simulink model "Colin_C_1_2020b"  (Simulink 10.3)
settings: Solver=ode45  StartTime=0.0  StopTime=5  RelTol=1e-3  AbsTol=1e-4
undefined symbols (not defined in the file or in its folder): C3, pendubot_eqt, Ts
libraries: simulink x4, SignalEditorBlockLib x1
Description:
  | Non-linear mathematical model of pendubot electro-mechanical system (underactuated pendulum system).
settings Model: Creator=Hynek Prochazka  LastModifiedBy=Colin  ExtModeTrigMode=oneshot  ExtModeArmWhenConnect=off
settings SolverCC: AutoScaleAbsTol=off
settings DataIOCC: SaveOutput=off
settings OptimizationCC: BlockReduction=off  BooleanDataType=off
settings DebuggingCC: SaveWithParameterizedLinksMsg=none  SignalResolutionControl=TryResolveAllWithWarning  MultiTaskDSMMsg=warning  MultiTaskCondExecSysMsg=none
settings HardwareCC: TargetUnknown=on
settings RTWCC: TemplateMakefile=grt_unix.tmf
settings ConfigComp: CovSFcnEnable=off

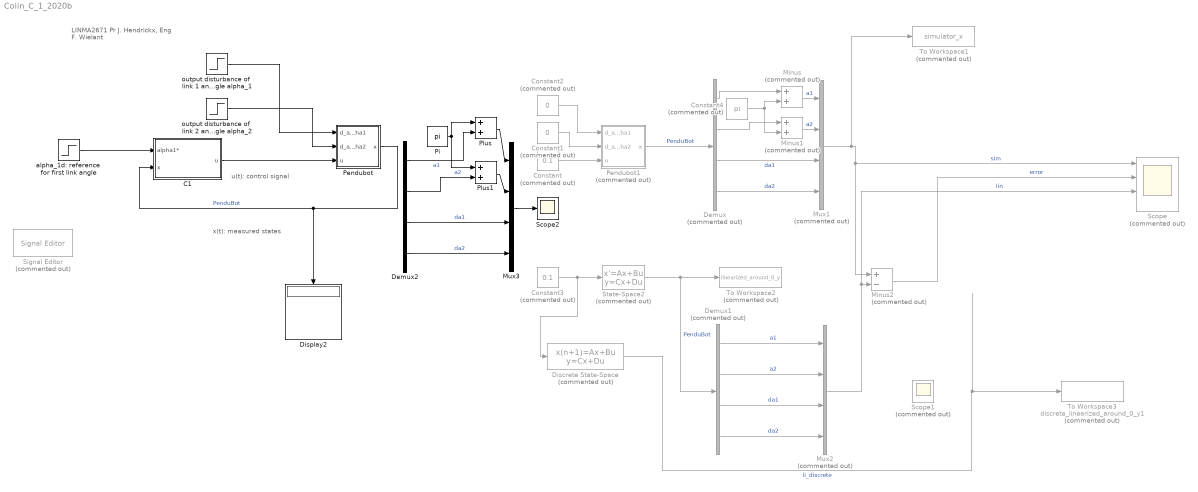
== system Colin_C_1_2020b ==
  note: u(t):
      | control signal
  note: x(t): measured states
  note: LINMA2671
      | Pr J. Hendrickx, Eng F. Wielant
  C1 : Subsystem
  Constant : Constant  Commented=on  Value=0.1
  Constant1 : Constant  Commented=on  Value=0
  Constant2 : Constant  Commented=on  Value=0
  Constant3 : Constant  Commented=on  Value=0.1
  Constant4 : Constant  Commented=on  Value=pi
  Demux : Demux  Commented=on
      settings: DisplayOption=none
  Demux1 : Demux  Commented=on
      settings: DisplayOption=none
  Demux2 : Demux
      settings: DisplayOption=none
  Discrete State-Space : DiscreteStateSpace  Commented=on  A=[0.9993,0.0004,0.004,0;0.0014,0.9987,0,0.004;-0.3693,0.2122,0.9993,0.0004;0.7023,-0.6366,0.0014,0.9987]  B=[0.0004;-0.0007;0.1859;-0.3535]  C=eye(4)  D=[0;0;0;0]  SampleTime=Ts
  Display2 : Display
  Minus : Sum  Commented=on
  Minus1 : Sum  Commented=on
  Minus2 : Sum  Commented=on  Inputs=+-
  Mux1 : Mux  Commented=on
  Mux2 : Mux  Commented=on
  Mux3 : Mux
  Pendubot : Subsystem  mask(Pendubot){x10=0, x20=0, x30=0, x40=0, Ts=Ts}
      mask prompts: x10 "Initial angle of link 1:"; x20 "Initial angular speed for link 1 :"; x30 "Initial angle of link 2 :"; x40 "Initial angular speed for link 2 :"; Ts "Sampling time [s] :"
      mask help: Initial conditions (initial state)
      mask Display:
      | plot(0.1*[1 9],0.1*[1 1])
      | plot(0.1*[1.5 1.5 8.5 8.5],0.1*[1 4 4 1])
      | plot(0.1*[5.2 8.2],0.1*[1 5])
      | plot(0.1*[4.8 7.8],0.1*[1 5])
      | plot(0.1*[7.8 5.8],0.1*[5 9.5])
      | plot(0.1*[8.2 6.2],0.1*[5 9.5])
  Pendubot1 : Subsystem  Commented=on  mask(Pendubot){x10=4*pi/5, x20=0, x30=pi, x40=0, Ts=Ts}
      mask prompts: x10 "Initial angle of link 1:"; x20 "Initial angular speed for link 1 :"; x30 "Initial angle of link 2 :"; x40 "Initial angular speed for link 2 :"; Ts "Sampling time [s] :"
      mask help: Initial conditions (initial state)
      mask Display:
      | plot(0.1*[1 9],0.1*[1 1])
      | plot(0.1*[1.5 1.5 8.5 8.5],0.1*[1 4 4 1])
      | plot(0.1*[5.2 8.2],0.1*[1 5])
      | plot(0.1*[4.8 7.8],0.1*[1 5])
      | plot(0.1*[7.8 5.8],0.1*[5 9.5])
      | plot(0.1*[8.2 6.2],0.1*[5 9.5])
  Pi : Constant  Value=pi  OutDataTypeStr=Inherit: Inherit via back propagation
  Plus : Sum
  Plus1 : Sum
  Scope : Scope  Commented=on  NumInputPorts=4
  Scope1 : Scope  Commented=on
  Scope2 : Scope
  Signal Editor : SignalEditorBlockLib/Signal Editor  Commented=on  FileName=untitled.mat  ActiveScenario=Scenario  ActiveSignal=Signal 1  IsBus=off  OutputBusObjectStr=Bus: BusObject  SampleTime=0  Interpolate=off  ZeroCross=off  OutputAfterFinalValue=Setting to zero  Unit=inherit  PreserveSignalName=on
  State-Space2 : StateSpace  Commented=on  A=[0,0,1,0;0,0,0,1;57.9843,-34.6580,0,0;-87.489,105.4244,0,0]  B=[0;0;40.9835;-70.8893]  C=eye(4)  D=[0;0;0;0]  InitialCondition=[0;0;0;0]
  To Workspace1 : ToWorkspace  Commented=on  VariableName=simulator_x  SaveFormat=Timeseries  SampleTime=Ts
  To Workspace2 : ToWorkspace  Commented=on  VariableName=linearized_around_0_y  SaveFormat=Timeseries  SampleTime=Ts
  To Workspace3 : ToWorkspace  Commented=on  VariableName=discrete_linearized_around_0_y1  SaveFormat=Timeseries  SampleTime=Ts
  "alpha_1d: reference  for first link angle " : Step  Time=2  After=4*pi/5  SampleTime=Ts
  output disturbance of  link 1 angle alpha_1 : Step  Time=5  After=0  SampleTime=Ts
  output disturbance of  link 2 angle alpha_2 : Step  Time=2  After=0  SampleTime=Ts
  wires:
  Pendubot/1(x) -> Display2/1, C1/2(x)  "PenduBot"
  C1/1(u) -> Pendubot/3(u)
  Constant/1 -> Pendubot1/3(u)
  Constant2/1 -> Pendubot1/1(d_alpha1)
  Constant1/1 -> Pendubot1/2(d_alpha2)
  Pendubot1/1(x) -> Demux/1  "PenduBot"
  Constant3/1 -> State-Space2/1, Discrete State-Space/1
  Minus/1 -> Mux1/1  "a1"
  Demux/1 -> Minus/1
  Constant4/1 -> Minus1/2, Minus/2
  Minus1/1 -> Mux1/2  "a2"
  Demux/2 -> Minus1/1
  Demux/3 -> Mux1/3  "da1"
  Demux/4 -> Mux1/4  "da2"
  Mux1/1 -> To Workspace1/1, Minus2/1, Scope/1  "sim"
  Demux1/2 -> Mux2/2  "a2"
  Demux1/1 -> Mux2/1  "a1"
  State-Space2/1 -> Demux1/1, To Workspace2/1  "PenduBot"
  Demux1/4 -> Mux2/4  "da2"
  Mux2/1 -> Minus2/2, Scope/3  "lin"
  Demux1/3 -> Mux2/3  "da1"
  Minus2/1 -> Scope/2  "error"
  Discrete State-Space/1 -> To Workspace3/1  "li_discrete"
  output disturbance of  link 1 angle alpha_1/1 -> Pendubot/1(d_alpha1)
  output disturbance of  link 2 angle alpha_2/1 -> Pendubot/2(d_alpha2)
  "alpha_1d: reference  for first link angle "/1 -> C1/1(alpha1*)
  Demux2/3 -> Mux3/3  "da1"
  Demux2/2 -> Plus1/2  "a2"
  Demux2/4 -> Mux3/4  "da2"
  Demux2/1 -> Plus/2  "a1"
  Mux3/1 -> Scope2/1
  Plus/1 -> Mux3/1
  Pi/1 -> Plus1/1, Plus/1
  Plus1/1 -> Mux3/2

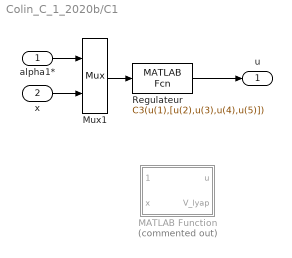
== system Colin_C_1_2020b/C1 ==
  alpha1* : Inport
  x : Inport  Port=2
  MATLAB Function : MATLAB Function  Commented=on  TreatAsAtomicUnit=on
  Mux1 : Mux  Inputs=2
  Regulateur : MATLABFcn  MATLABFcn=C3(u(1),[u(2),u(3),u(4),u(5)])
  u : Outport
  wires:
  Mux1/1 -> Regulateur/1
  alpha1*/1 -> Mux1/1
  x/1 -> Mux1/2
  Regulateur/1 -> u/1

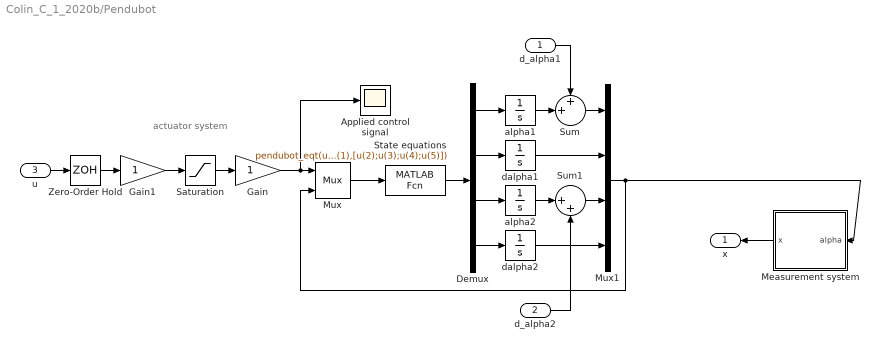
== system Colin_C_1_2020b/Pendubot ==
  note: actuator system
  d_alpha1 : Inport
  d_alpha2 : Inport  Port=2
  u : Inport  Port=3
  Applied control signal : Scope
  Demux : Demux
      settings: DisplayOption=none
  Gain : Gain  SaturateOnIntegerOverflow=on  OutDataTypeStr=Inherit: Same as input  ParamDataTypeStr=Inherit: Same as input
  Gain1 : Gain  SaturateOnIntegerOverflow=on  OutDataTypeStr=Inherit: Same as input  ParamDataTypeStr=Inherit: Same as input
  Measurement system : Subsystem
  Mux : Mux  Inputs=2
  Mux1 : Mux
  Saturation : Saturate  UpperLimit=10  LowerLimit=-10
  State equations : MATLABFcn  MATLABFcn=pendubot_eqt(u(1),[u(2);u(3);u(4);u(5)])  OutputDimensions=4
  Sum : Sum  Inputs=++|  InputSameDT=on  SaturateOnIntegerOverflow=on  OutDataTypeStr=Inherit: Same as first input
  Sum1 : Sum  Inputs=|++  InputSameDT=on  SaturateOnIntegerOverflow=on  OutDataTypeStr=Inherit: Same as first input
  Zero-Order Hold : ZeroOrderHold  SampleTime=Ts
  alpha1 : Integrator  InitialCondition=x10
  alpha2 : Integrator  InitialCondition=x30
  dalpha1 : Integrator  InitialCondition=x20
  dalpha2 : Integrator  InitialCondition=x40
  x : Outport
  wires:
  u/1 -> Zero-Order Hold/1
  State equations/1 -> Demux/1
  Mux/1 -> State equations/1
  Saturation/1 -> Gain/1
  Zero-Order Hold/1 -> Gain1/1
  Gain1/1 -> Saturation/1
  Gain/1 -> Mux/1, Applied control signal/1
  Mux1/1 -> Mux/2, Measurement system/1(alpha)
  dalpha2/1 -> Mux1/4
  Demux/1 -> alpha1/1
  Demux/2 -> dalpha1/1
  Demux/3 -> alpha2/1
  Demux/4 -> dalpha2/1
  Sum/1 -> Mux1/1
  Sum1/1 -> Mux1/3
  dalpha1/1 -> Mux1/2
  alpha1/1 -> Sum/2
  d_alpha1/1 -> Sum/1
  alpha2/1 -> Sum1/1
  d_alpha2/1 -> Sum1/2
  Measurement system/1(x) -> x/1

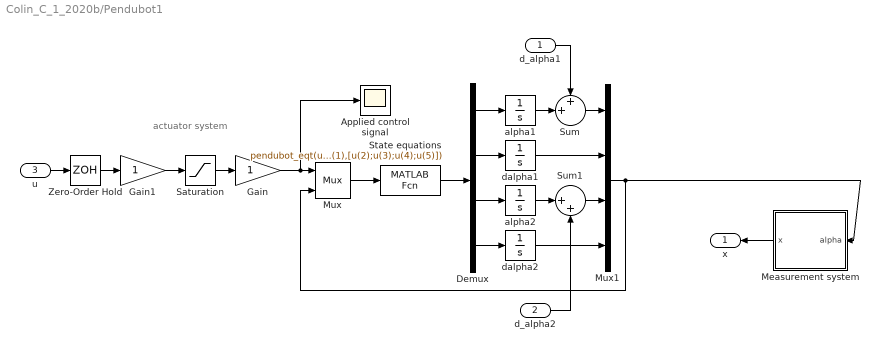
== system Colin_C_1_2020b/Pendubot1 ==
  note: actuator system
  d_alpha1 : Inport
  d_alpha2 : Inport  Port=2
  u : Inport  Port=3
  Applied control signal : Scope
  Demux : Demux
      settings: DisplayOption=none
  Gain : Gain  SaturateOnIntegerOverflow=on  OutDataTypeStr=Inherit: Same as input  ParamDataTypeStr=Inherit: Same as input
  Gain1 : Gain  SaturateOnIntegerOverflow=on  OutDataTypeStr=Inherit: Same as input  ParamDataTypeStr=Inherit: Same as input
  Measurement system : Subsystem
  Mux : Mux  Inputs=2
  Mux1 : Mux
  Saturation : Saturate  UpperLimit=10  LowerLimit=-10
  State equations : MATLABFcn  MATLABFcn=pendubot_eqt(u(1),[u(2);u(3);u(4);u(5)])  OutputDimensions=4
  Sum : Sum  Inputs=++|  InputSameDT=on  SaturateOnIntegerOverflow=on  OutDataTypeStr=Inherit: Same as first input
  Sum1 : Sum  Inputs=|++  InputSameDT=on  SaturateOnIntegerOverflow=on  OutDataTypeStr=Inherit: Same as first input
  Zero-Order Hold : ZeroOrderHold  SampleTime=Ts
  alpha1 : Integrator  InitialCondition=x10
  alpha2 : Integrator  InitialCondition=x30
  dalpha1 : Integrator  InitialCondition=x20
  dalpha2 : Integrator  InitialCondition=x40
  x : Outport
  wires:
  u/1 -> Zero-Order Hold/1
  State equations/1 -> Demux/1
  Mux/1 -> State equations/1
  Saturation/1 -> Gain/1
  Zero-Order Hold/1 -> Gain1/1
  Gain1/1 -> Saturation/1
  Gain/1 -> Mux/1, Applied control signal/1
  Mux1/1 -> Mux/2, Measurement system/1(alpha)
  dalpha2/1 -> Mux1/4
  Demux/1 -> alpha1/1
  Demux/2 -> dalpha1/1
  Demux/3 -> alpha2/1
  Demux/4 -> dalpha2/1
  Sum/1 -> Mux1/1
  Sum1/1 -> Mux1/3
  dalpha1/1 -> Mux1/2
  alpha1/1 -> Sum/2
  d_alpha1/1 -> Sum/1
  alpha2/1 -> Sum1/1
  d_alpha2/1 -> Sum1/2
  Measurement system/1(x) -> x/1

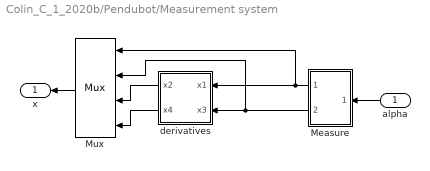
== system Colin_C_1_2020b/Pendubot/Measurement system ==
  alpha : Inport
  Measure : Subsystem
  Mux : Mux
  derivatives : Subsystem
  x : Outport
  wires:
  derivatives/2(x4) -> Mux/4
  Mux/1 -> x/1
  Measure/1(xm(1)) -> derivatives/1(x1), Mux/1
  alpha/1 -> Measure/1(alpha)
  Measure/2(xm(1)1) -> derivatives/2(x3), Mux/2
  derivatives/1(x2) -> Mux/3

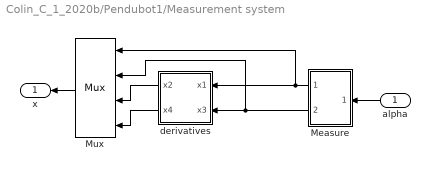
== system Colin_C_1_2020b/Pendubot1/Measurement system ==
  alpha : Inport
  Measure : Subsystem
  Mux : Mux
  derivatives : Subsystem
  x : Outport
  wires:
  derivatives/2(x4) -> Mux/4
  Mux/1 -> x/1
  Measure/1(xm(1)) -> derivatives/1(x1), Mux/1
  alpha/1 -> Measure/1(alpha)
  Measure/2(xm(1)1) -> derivatives/2(x3), Mux/2
  derivatives/1(x2) -> Mux/3

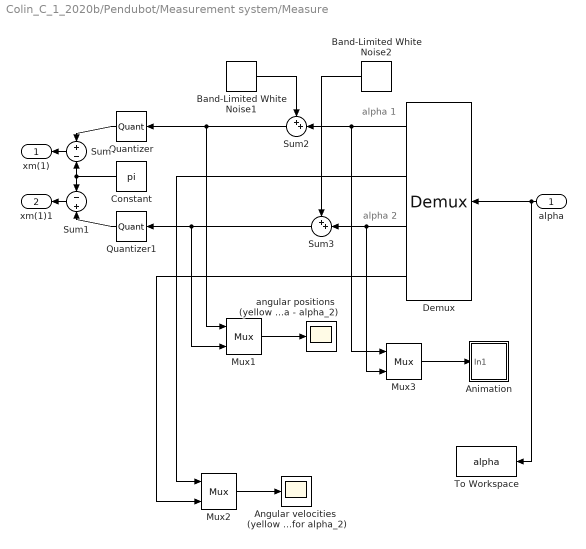
== system Colin_C_1_2020b/Pendubot/Measurement system/Measure ==
  note: alpha 1
  note: alpha 2
  alpha : Inport
  "Angular velocities  (yellow - for alpha_1,  magenta - for alpha_2) " : Scope
  Animation : Subsystem  mask(Animation Block){ts=10*0.003}
      mask prompts: ts "Sample time:"
      mask Display: plot([.1,.9],[.9,.9],[.5,.2],[.9,.25],[.475,.475,.525,.525,.475],[.875,.925,.925,.875,.875])
  Band-Limited White Noise1 : simulink/Sources/Band-Limited White Noise  Cov=[1e-8]  Ts=Ts  seed=[23341]
  Band-Limited White Noise2 : simulink/Sources/Band-Limited White Noise  Cov=[1e-7]  Ts=Ts  seed=[32214]
  Constant : Constant  Value=pi
  Demux : Demux
      settings: DisplayOption=none
  Mux1 : Mux  Inputs=2
  Mux2 : Mux  Inputs=2
  Mux3 : Mux  Inputs=2
  Quantizer : Quantizer  QuantizationInterval=2*pi/5000
  Quantizer1 : Quantizer  QuantizationInterval=2*pi/5000
  Sum : Sum  Inputs=+-  InputSameDT=on  SaturateOnIntegerOverflow=on  OutDataTypeStr=Inherit: Same as first input
  Sum1 : Sum  Inputs=-+  InputSameDT=on  SaturateOnIntegerOverflow=on  OutDataTypeStr=Inherit: Same as first input
  Sum2 : Sum  Inputs=++|  InputSameDT=on  SaturateOnIntegerOverflow=on  OutDataTypeStr=Inherit: Same as first input
  Sum3 : Sum  Inputs=++|  InputSameDT=on  SaturateOnIntegerOverflow=on  OutDataTypeStr=Inherit: Same as first input
  To Workspace : ToWorkspace  VariableName=alpha  SampleTime=Ts
  "angular positions  (yellow - alpha_1,  magenta - alpha_2)" : Scope
  xm(1) : Outport  Tag=alpha1
  xm(1)1 : Outport  Port=2
  wires:
  alpha/1 -> To Workspace/1, Demux/1
  Demux/2 -> Mux2/1
  Demux/4 -> Mux2/2
  Mux2/1 -> "Angular velocities  (yellow - for alpha_1,  magenta - for alpha_2) "/1
  Sum/1 -> xm(1)/1
  Quantizer/1 -> Sum/1
  Sum1/1 -> xm(1)1/1
  Quantizer1/1 -> Sum1/2
  Constant/1 -> Sum/2, Sum1/1
  Band-Limited White Noise1/1 -> Sum2/1
  Band-Limited White Noise2/1 -> Sum3/1
  Sum2/1 -> Quantizer/1, Mux1/1
  Sum3/1 -> Quantizer1/1, Mux1/2
  Mux1/1 -> "angular positions  (yellow - alpha_1,  magenta - alpha_2)"/1
  Demux/1 -> Sum2/2, Mux3/1
  Demux/3 -> Sum3/2, Mux3/2
  Mux3/1 -> Animation/1(In1)

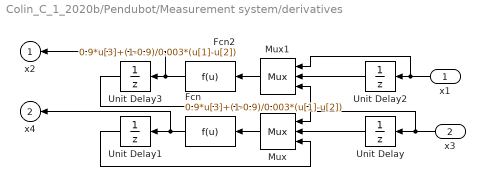
== system Colin_C_1_2020b/Pendubot/Measurement system/derivatives ==
  x1 : Inport
  x3 : Inport  Port=2
  Fcn : Fcn  Expr=0.9*u[3]+(1-0.9)/0.003*(u[1]-u[2])
  Fcn2 : Fcn  Expr=0.9*u[3]+(1-0.9)/0.003*(u[1]-u[2])
  Mux : Mux  Inputs=3
  Mux1 : Mux  Inputs=3
  Unit Delay{,1..3} (4 alike) : UnitDelay  SampleTime=Ts  HasFrameUpgradeWarning=on
  x2 : Outport
  x4 : Outport  Port=2
  wires:
  Unit Delay/1 -> Mux/2
  Mux/1 -> Fcn/1
  Unit Delay1/1 -> Mux/3
  Fcn/1 -> Unit Delay1/1, x4/1
  x3/1 -> Unit Delay/1, Mux/1
  Unit Delay2/1 -> Mux1/2
  Mux1/1 -> Fcn2/1
  Unit Delay3/1 -> Mux1/3
  x1/1 -> Unit Delay2/1, Mux1/1
  Fcn2/1 -> Unit Delay3/1, x2/1

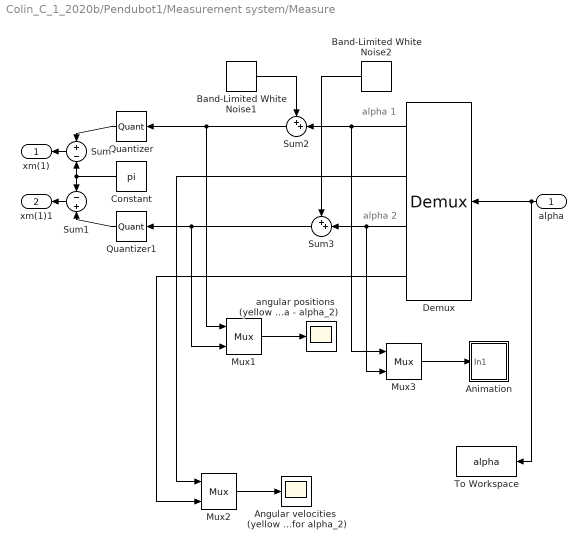
== system Colin_C_1_2020b/Pendubot1/Measurement system/Measure ==
  note: alpha 1
  note: alpha 2
  alpha : Inport
  "Angular velocities  (yellow - for alpha_1,  magenta - for alpha_2) " : Scope
  Animation : Subsystem  mask(Animation Block){ts=10*0.003}
      mask prompts: ts "Sample time:"
      mask Display: plot([.1,.9],[.9,.9],[.5,.2],[.9,.25],[.475,.475,.525,.525,.475],[.875,.925,.925,.875,.875])
  Band-Limited White Noise1 : simulink/Sources/Band-Limited White Noise  Cov=[1e-8]  Ts=Ts  seed=[23341]
  Band-Limited White Noise2 : simulink/Sources/Band-Limited White Noise  Cov=[1e-7]  Ts=Ts  seed=[32214]
  Constant : Constant  Value=pi
  Demux : Demux
      settings: DisplayOption=none
  Mux1 : Mux  Inputs=2
  Mux2 : Mux  Inputs=2
  Mux3 : Mux  Inputs=2
  Quantizer : Quantizer  QuantizationInterval=2*pi/5000
  Quantizer1 : Quantizer  QuantizationInterval=2*pi/5000
  Sum : Sum  Inputs=+-  InputSameDT=on  SaturateOnIntegerOverflow=on  OutDataTypeStr=Inherit: Same as first input
  Sum1 : Sum  Inputs=-+  InputSameDT=on  SaturateOnIntegerOverflow=on  OutDataTypeStr=Inherit: Same as first input
  Sum2 : Sum  Inputs=++|  InputSameDT=on  SaturateOnIntegerOverflow=on  OutDataTypeStr=Inherit: Same as first input
  Sum3 : Sum  Inputs=++|  InputSameDT=on  SaturateOnIntegerOverflow=on  OutDataTypeStr=Inherit: Same as first input
  To Workspace : ToWorkspace  VariableName=alpha  SampleTime=Ts
  "angular positions  (yellow - alpha_1,  magenta - alpha_2)" : Scope
  xm(1) : Outport  Tag=alpha1
  xm(1)1 : Outport  Port=2
  wires:
  alpha/1 -> To Workspace/1, Demux/1
  Demux/2 -> Mux2/1
  Demux/4 -> Mux2/2
  Mux2/1 -> "Angular velocities  (yellow - for alpha_1,  magenta - for alpha_2) "/1
  Sum/1 -> xm(1)/1
  Quantizer/1 -> Sum/1
  Sum1/1 -> xm(1)1/1
  Quantizer1/1 -> Sum1/2
  Constant/1 -> Sum/2, Sum1/1
  Band-Limited White Noise1/1 -> Sum2/1
  Band-Limited White Noise2/1 -> Sum3/1
  Sum2/1 -> Quantizer/1, Mux1/1
  Sum3/1 -> Quantizer1/1, Mux1/2
  Mux1/1 -> "angular positions  (yellow - alpha_1,  magenta - alpha_2)"/1
  Demux/1 -> Sum2/2, Mux3/1
  Demux/3 -> Sum3/2, Mux3/2
  Mux3/1 -> Animation/1(In1)

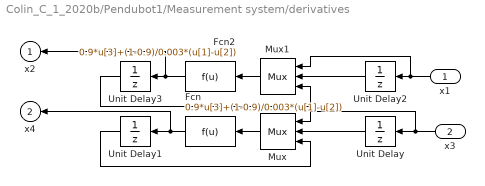
== system Colin_C_1_2020b/Pendubot1/Measurement system/derivatives ==
  x1 : Inport
  x3 : Inport  Port=2
  Fcn : Fcn  Expr=0.9*u[3]+(1-0.9)/0.003*(u[1]-u[2])
  Fcn2 : Fcn  Expr=0.9*u[3]+(1-0.9)/0.003*(u[1]-u[2])
  Mux : Mux  Inputs=3
  Mux1 : Mux  Inputs=3
  Unit Delay{,1..3} (4 alike) : UnitDelay  SampleTime=Ts  HasFrameUpgradeWarning=on
  x2 : Outport
  x4 : Outport  Port=2
  wires:
  Unit Delay/1 -> Mux/2
  Mux/1 -> Fcn/1
  Unit Delay1/1 -> Mux/3
  Fcn/1 -> Unit Delay1/1, x4/1
  x3/1 -> Unit Delay/1, Mux/1
  Unit Delay2/1 -> Mux1/2
  Mux1/1 -> Fcn2/1
  Unit Delay3/1 -> Mux1/3
  x1/1 -> Unit Delay2/1, Mux1/1
  Fcn2/1 -> Unit Delay3/1, x2/1

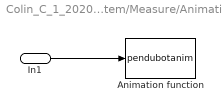
== system Colin_C_1_2020b/Pendubot/Measurement system/Measure/Animation ==
  In1 : Inport
  Animation function : S-Function  FunctionName=pendubotanim  Parameters=ts  SFunctionDeploymentMode=off  EnableBusSupport=off
      settings: DeleteFcn=if ~isempty(findobj('type','figure','name','simppend Animation'));close('simppend Animation'); end;
  wires:
  In1/1 -> Animation function/1

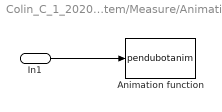
== system Colin_C_1_2020b/Pendubot1/Measurement system/Measure/Animation ==
  In1 : Inport
  Animation function : S-Function  FunctionName=pendubotanim  Parameters=ts  SFunctionDeploymentMode=off  EnableBusSupport=off
      settings: DeleteFcn=if ~isempty(findobj('type','figure','name','simppend Animation'));close('simppend Animation'); end;
  wires:
  In1/1 -> Animation function/1

== matlab function C1/MATLAB Function ==
  data: alpha1r input double; u output double; x input double; V_lyap output double
function [u, V_lyap] = pendulumNonLinear(alpha1r,x)
%UNTITLED Summary of this function goes here
%   Detailed explanation goes here
    alpha1 = x(1);
    alpha2 = x(2);
    dalpha1 = x(3);
    dalpha2 = x(4);

    p1 = 0.0148; p2 = 0.0051; p3 = 0.0046; p4 = 0.1003; p5 = 0.0303;
    g = 9.81;
    E_ref = (p4 + p5) * g;

    % Mass matrix M(alpha)
    M = [p1 + p2 + 2*p3*cos(alpha2 - alpha1), p2 + p3*cos(alpha2 - alpha1);
         p2 + p3*cos(alpha2 - alpha1), p2];

    % Potential energy V
    V = -p4*g*cos(alpha1) - p5*g*cos(alpha2);

    % Kinetic energy T
    T = 0.5 * [dalpha1 dalpha2] * M * [dalpha1; dalpha2];

    % Total energy
    E = T + V;

    % Lyapunov Function (Energy-based)
    V_lyap = E;
    k_p = 0.5;
    k_d = 0.1;
    % Derivative of the Lyapunov Function
    dV_lyap = [dalpha1; dalpha2]' * (0.5 * M * [dalpha1; dalpha2] + [p4*g*sin(alpha1); p5*g*sin(alpha2)]);

    corr_x = [x(1) ; x(2) ; x(3) ; x(4)];
    % Control Law for Swing-Up using PD controller
    u = -k_p * corr_x;

end
